simulink model "flood_drainage_system_2_R2025a"  (R2025a)
settings: Solver=VariableStepAuto  StartTime=0.0  StopTime=inf  FixedStep=1  RelTol=1e-3
undefined symbols (not defined in the file): DiscIntNeverNeededParam
libraries: simulink x15
(part 3 of 3)

== matlab function flood_drainage_system_2_R2025a/Sensor Fusion/MATLAB Function3 ==
  data: noisy_input input; x_est output
function x_est = kalmanFilter(noisy_input)

persistent x P
if isempty(x), x = noisy_input; end
if isempty(P), P = 1; end


Q = 1e-3;   % process noise covariance
R = 1e-4;   % measurement noise covariance

% prediction
x_pred = x;
P_pred = P + Q;

% update
K = P_pred / (P_pred + R);
x = x_pred + K*(noisy_input - x_pred);
P = (1 - K)*P_pred;

x_est = x;
